simulink model "s32k344_mcb_sensorless_s32ct"  (R2024b)
settings: Solver=FixedStepAuto  StartTime=0.0  StopTime=20  RelTol=1e-3  EnableMultiTasking=on
PreLoadFcn:
  | % NXP_MBDT_S32K3 callback: DO NOT REMOVE
  | mbd_s32k3.common.nxp.model_callbacks.preLoadFcn();
  | 
  | s32k344Data;
  | mcbSensorlessData;
PostLoadFcn:
  | % NXP_MBDT_S32K3 callback: DO NOT REMOVE
  | mbd_s32k3.common.nxp.model_callbacks.postLoadFcn();
InitFcn:
  | % NXP_MBDT_S32K3 callback: DO NOT REMOVE
  | mbd_s32k3.common.nxp.model_callbacks.initFcn();
values from neighbouring files (symbols this model uses):
  PWM_DutyScale = 32768    [s32k344Data.m]
  PWM_Period = 8000    [s32k344Data.m]
  Ts_motor = T_pwm    (= 5e-05)    [s32k344Data.m]
  Ts_SerialIn = 0.1    [s32k344Data.m]
  Ts_SerialOut = 0.01    [s32k344Data.m]
  Ts_SysControl = 0.1    [mcbSensorlessData.m]
undefined symbols (not defined in the file or in its folder): inverter, LogicOutputId, pmsm, Value
libraries: mbd_s32k3_io_library x14, mbd_s32k3_cdd_library x4, simulink x4, mbd_s32k3_isr_library x1, mbd_s32k3_utility_library x1
(part 2 of 3)

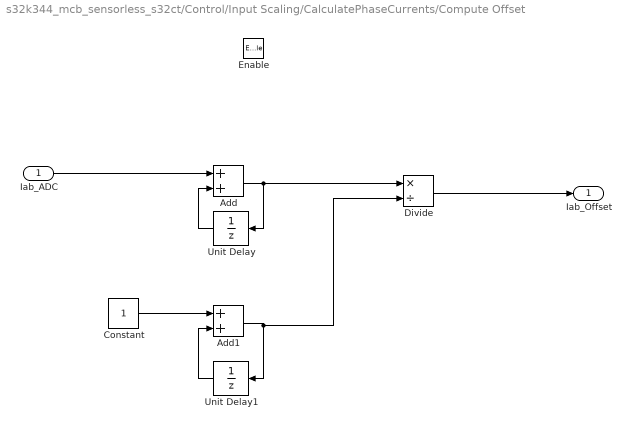
== system s32k344_mcb_sensorless_s32ct/Control/Input Scaling/CalculatePhaseCurrents/Compute Offset ==
  Iab_ADC : Inport
  Enable : EnablePort
  Add : Sum  RndMeth=Simplest  OutDataTypeStr=Inherit: Same as first input
  Add1 : Sum  RndMeth=Simplest  OutDataTypeStr=Inherit: Same as first input
  Constant : Constant  OutDataTypeStr=uint32  SampleTime=-1
  Divide : Product  Inputs=*/  RndMeth=Simplest  OutDataTypeStr=Inherit: Same as first input
  Unit Delay : UnitDelay  SampleTime=-1  HasFrameUpgradeWarning=on
  Unit Delay1 : UnitDelay  SampleTime=-1  HasFrameUpgradeWarning=on
  Iab_Offset : Outport
  wires:
  Iab_ADC/1 -> Add/1
  Unit Delay/1 -> Add/2
  Add/1 -> Divide/1, Unit Delay/1
  Constant/1 -> Add1/1
  Unit Delay1/1 -> Add1/2
  Add1/1 -> Divide/2, Unit Delay1/1
  Divide/1 -> Iab_Offset/1

== system s32k344_mcb_sensorless_s32ct/Control/SerialReceive/Variant Subsystem/CodeGeneration ==
  Constant : Constant  Value=8  OutDataTypeStr=Inherit: Inherit via back propagation
  Terminator : Terminator
  Uart : mbd_s32k3_cdd_library/Uart  api_func=Uart_AsyncReceive  channel=UartChannel_6  baudrate=UART_BAUDRATE_1200  transfer_type=UART_SEND  timeout=1  text=<binary blob, 3405 chars, not shown>
      settings: SourceProductName=CDD Blocks
  Data : Outport
  wires:
  Constant/1 -> Uart/1
  Uart/1 -> Data/1
  Uart/2 -> Terminator/1

== system s32k344_mcb_sensorless_s32ct/Control/SerialReceive/Variant Subsystem/Simulation ==
  Ground : Ground
  Data : Outport
  wires:
  Ground/1 -> Data/1

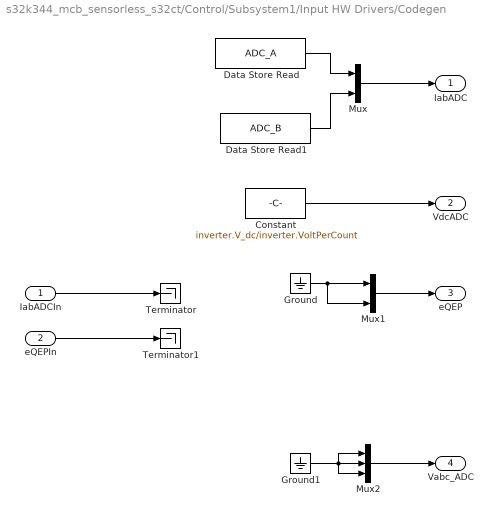
== system s32k344_mcb_sensorless_s32ct/Control/Subsystem1/Input HW Drivers/Codegen ==
  IabADCIn : Inport
  eQEPIn : Inport  Port=2
  Constant : Constant  Value=inverter.V_dc/inverter.VoltPerCount  OutDataTypeStr=uint16  SampleTime=-1
  Data Store Read : DataStoreRead  DataStoreName=ADC_A  IndexOptions=Index vector (dialog)  Indices=1  OutputSizes=1
  Data Store Read1 : DataStoreRead  DataStoreName=ADC_B  IndexOptions=Index vector (dialog)  Indices=1  OutputSizes=1
  Ground : Ground
  Ground1 : Ground
  Mux : Mux  Inputs=2
  Mux1 : Mux  Inputs=2
  Mux2 : Mux  Inputs=3
  Terminator : Terminator
  Terminator1 : Terminator
  IabADC : Outport
  VdcADC : Outport  Port=2
  eQEP : Outport  Port=3
  Vabc_ADC : Outport  Port=4
  wires:
  Ground/1 -> Mux1/2, Mux1/1
  Mux/1 -> IabADC/1
  Data Store Read1/1 -> Mux/2
  Constant/1 -> VdcADC/1
  Data Store Read/1 -> Mux/1
  Mux1/1 -> eQEP/1
  IabADCIn/1 -> Terminator/1
  eQEPIn/1 -> Terminator1/1
  Mux2/1 -> Vabc_ADC/1
  Ground1/1 -> Mux2/1, Mux2/3, Mux2/2

== system s32k344_mcb_sensorless_s32ct/Control/Subsystem1/Input HW Drivers/Sim ==
  IabADCIn : Inport
  eQEPIn : Inport  Port=2
  Constant : Constant  Value=inverter.V_dc/inverter.VoltPerCount  OutDataTypeStr=uint16  SampleTime=-1
  Ground : Ground
  IabADC : Outport
  VdcADC : Outport  Port=2
  Vabc_ADC : Outport  Port=3
  eQEP : Outport  Port=4
  wires:
  Constant/1 -> VdcADC/1
  Ground/1 -> Vabc_ADC/1
  IabADCIn/1 -> IabADC/1
  eQEPIn/1 -> eQEP/1

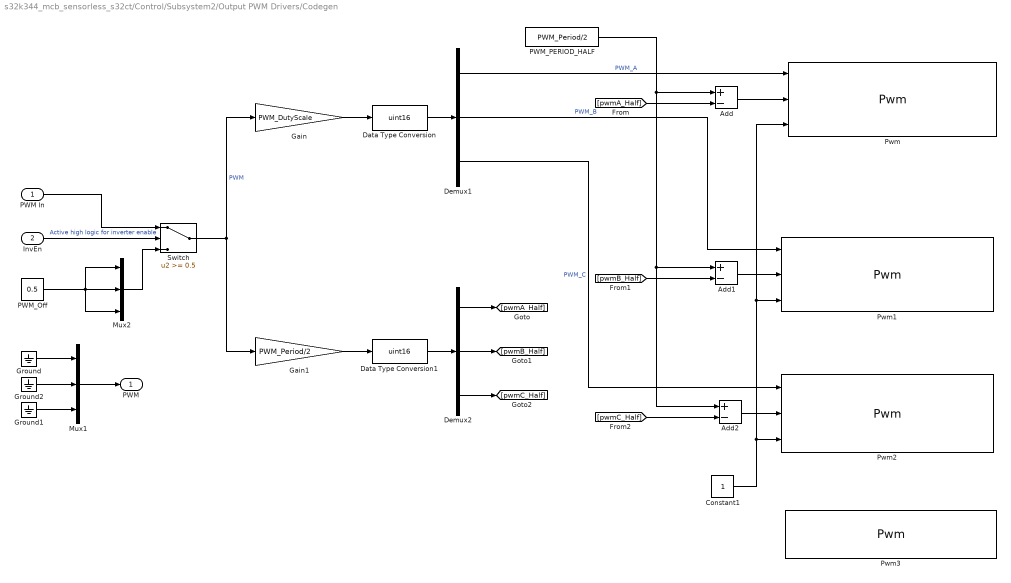
== system s32k344_mcb_sensorless_s32ct/Control/Subsystem2/Output PWM Drivers/Codegen ==
  PWM In : Inport
  InvEn : Inport  Port=2
  Add : Sum  Inputs=+-  OutDataTypeStr=uint16
  Add1 : Sum  Inputs=+-  OutDataTypeStr=uint16
  Add2 : Sum  Inputs=+-  OutDataTypeStr=uint16
  Constant1 : Constant  OutDataTypeStr=boolean  SampleTime=-1
  Data Type Conversion : DataTypeConversion  OutDataTypeStr=uint16  SaturateOnIntegerOverflow=off  RndMeth=Floor
  Data Type Conversion1 : DataTypeConversion  OutDataTypeStr=uint16  SaturateOnIntegerOverflow=off  RndMeth=Floor
  Demux1 : Demux  Outputs=3
  Demux2 : Demux  Outputs=3
  Gain : Gain  Gain=PWM_DutyScale  OutDataTypeStr=single
  Gain1 : Gain  Gain=PWM_Period/2  OutDataTypeStr=single
  Ground : Ground
  Ground1 : Ground
  Ground2 : Ground
  Mux1 : Mux  Inputs=3
  Mux2 : Mux  Inputs=3
  PWM_Off : Constant  Value=0.5  OutDataTypeStr=single
  PWM_PERIOD_HALF : Constant  Value=PWM_Period/2  OutDataTypeStr=uint16
  Pwm : mbd_s32k3_io_library/Pwm  api_func=Pwm_SetDutyPhaseShift  channel=PwmChannel_0  notification=PWM_RISING_EDGE  moduleId=PWM_EMIOS_INSTANCE_0  prescalerType=PWM_PRIMARY_PRESCALER  fault=PWM_FLEXPWM_0_FAULT_INPUT_0  text=|
      | CommonPublishedInformation - CommonPublishedInformation Pwm 
      | CommonPublishedInformation/ArReleaseMajorVersion - 4 
      | CommonPublishedInformation/ArReleaseMinorVersion - 7 
      | CommonPublishedInformation/ArReleaseRevisionVersion - 0 
      | CommonPublishedInformation/ModuleId - 121 
      | CommonPublishedInformation/SwMajorVersion - 4 
      | CommonPublishedInformation/SwMinorVersion - 0 
      | CommonPublishedInformation/SwPatchVersion - 0 
      | CommonPublishedInformation/VendorId - 43 
      | IMPLEMENTATION-CONFIG-VARIANT - VARIANT-POST-BUILD 
      | POST_BUILD_VARIANT_USED - true 
      | PwmChannel - PwmChannel_0 PwmChannel_1 PwmChannel_2 PwmChannel_3 
      | PwmChannel_0/Index - 0 
      | PwmChannel_0/PwmChannelId - 0 
      | PwmChannel_0/PwmDutycycleDefault - 16384 
      | PwmChannel_0/PwmHwChannel - /Pwm/Pwm/PwmChannelConfigSet/PwmEmios_0/PwmEmiosChannels_0 
      | PwmChannel_0/PwmIdleState - PWM_LOW 
      | PwmChannel_0/PwmMcuClockReferencePoint - /Mcu/Mcu/McuModuleConfiguration/McuClockSettingConfig_0/CORE_CLK 
      | PwmChannel_0/PwmPeriodDefault - 8000.0 
      | PwmChannel_0/PwmPeriodInTicks - true 
      | PwmChannel_0/PwmPolarity - PWM_HIGH 
      | PwmChannel_1/Index - 1 
      | PwmChannel_1/PwmChannelId - 1 
      | PwmChannel_1/PwmDutycycleDefault - 16384 
      | PwmChannel_1/PwmHwChannel - /Pwm/Pwm/PwmChannelConfigSet/PwmEmios_0/PwmEmiosChannels_1 
      | PwmChannel_1/PwmIdleState - PWM_LOW 
      | PwmChannel_1/PwmMcuClockReferencePoint - /Mcu/Mcu/McuModuleConfiguration/McuClockSettingConfig_0/CORE_CLK 
      | PwmChannel_1/PwmPeriodDefault - 8000.0 
      | PwmChannel_1/PwmPeriodInTicks - true 
      | PwmChannel_1/PwmPolarity - PWM_HIGH 
      | PwmChannel_2/Index - 2 
      | PwmChannel_2/PwmChannelId - 2 
      | PwmChannel_2/PwmDutycycleDefault - 16384 
      | PwmChannel_2/PwmHwChannel - /Pwm/Pwm/PwmChannelConfigSet/PwmEmios_0/PwmEmiosChannels_2 
      | PwmChannel_2/PwmIdleState - PWM_LOW 
      | PwmChannel_2/PwmMcuClockReferencePoint - /Mcu/Mcu/McuModuleConfiguration/McuClockSettingConfig_0/CORE_CLK 
      | PwmChannel_2/PwmPeriodDefault - 8000.0 
      | PwmChannel_2/PwmPeriodInTicks - true 
      | PwmChannel_2/PwmPolarity - PWM_HIGH 
      | PwmChannel_3/Index - 3 
      | PwmChannel_3/PwmChannelId - 3 
      | PwmChannel_3/PwmDutycycleDefault - 5 
      | PwmChannel_3/PwmHwChannel - /Pwm/Pwm/PwmChannelConfigSet/PwmEmios_0/PwmEmiosChannels_3 
      | PwmChannel_3/PwmIdleState - PWM_LOW 
      | PwmChannel_3/PwmMcuClockReferencePoint - /Mcu/Mcu/McuModuleConfiguration/McuClockSettingConfig_0/CORE_CLK 
      | PwmChannel_3/PwmPeriodDefault - 16000 
      | PwmChannel_3/PwmPeriodInTicks - true 
      | PwmChannel_3/PwmPolarity - PWM_HIGH 
      | PwmConfigurationOfOptApiServices - PwmConfigurationOfOptApiServices 
      | PwmConfigurationOfOptApiServices/PwmDeInitApi - false 
      | PwmConfigurationOfOptApiServices/PwmEmiosFastUpdateApi - true 
      | PwmConfigurationOfOptApiServices/PwmEnableMaskOutputs - false 
      | PwmConfigurationOfOptApiServices/PwmGetChannelStateApi - false 
      | PwmConfigurationOfOptApiServices/PwmGetOutputState - false 
      | PwmConfigurationOfOptApiServices/PwmSetChannelDeadTime - false 
      | PwmConfigurationOfOptApiServices/PwmSetChannelOutputApi - false 
      | PwmConfigurationOfOptApiServices/PwmSetCounterBusApi - false 
      | PwmConfigurationOfOptApiServices/PwmSetDutyCycle - true 
      | PwmConfigurationOfOptApiServices/PwmSetDutyCycle_NoUpdate - true 
      | PwmConfigurationOfOptApiServices/PwmSetDutyPhaseShift - true 
      | PwmConfigurationOfOptApiServices/PwmSetOutputToIdle - false 
      | PwmConfigurationOfOptApiServices/PwmSetPeriodAndDuty - false 
      | PwmConfigurationOfOptApiServices/PwmSetPeriodAndDuty_NoUpdate - false 
      | PwmConfigurationOfOptApiServices/PwmSetTriggerDelayApi - false 
      | PwmConfigurationOfOptApiServices/PwmVersionInfoApi - false 
      | PwmEmios - PwmEmios_0 
      | PwmEmios_0/Index - 0 
      | PwmEmios_0/PwmEmiosChannels - PwmEmiosChannels_0 PwmEmiosChannels_1 PwmEmiosChannels_2 PwmEmiosChannels_3 
      | PwmEmios_0/PwmEmiosChannels_0/EmiosChCounterBus - EMIOS_PWM_IP_BUS_BCD 
      | PwmEmios_0/PwmEmiosChannels_0/EmiosChDeadtime - 0 
      | PwmEmios_0/PwmEmiosChannels_0/EmiosChFlagGeneration - Trailing_Edge 
      | PwmEmios_0/PwmEmiosChannels_0/EmiosChFreeze - false 
      | PwmEmios_0/PwmEmiosChannels_0/EmiosChId - CH_1 
      | PwmEmios_0/PwmEmiosChannels_0/EmiosChInterrupt - EMIOS_PWM_IP_NOTIFICATION_DISABLED 
      | PwmEmios_0/PwmEmiosChannels_0/EmiosChMode - EMIOS_PWM_IP_MODE_OPWMB 
      | PwmEmios_0/PwmEmiosChannels_0/EmiosChOutputDisable - EMIOS_PWM_IP_OUTPUT_DISABLE_NONE 
      | PwmEmios_0/PwmEmiosChannels_0/EmiosChPhaseShift - 0 
      | PwmEmios_0/PwmEmiosChannels_0/EmiosChPrescaler - EMIOS_PWM_IP_CLOCK_DIV_1 
      | PwmEmios_0/PwmEmiosChannels_0/EmiosChPrescalerAlternate - EMIOS_PWM_IP_CLOCK_DIV_1 
      | PwmEmios_0/PwmEmiosChannels_0/EmiosChPrescalerSource - EMIOS_PWM_IP_PS_SRC_MODULE_CLOCK 
      | PwmEmios_0/PwmEmiosChannels_0/EmiosChTrigger - 0 
      | PwmEmios_0/PwmEmiosChannels_0/Index - 0 
      | PwmEmios_0/PwmEmiosChannels_0/PwmEmiosBusRef - /Mcl/Mcl/MclConfig/EmiosCommon_0/EmiosMclMasterBus_0 
      | PwmEmios_0/PwmEmiosChannels_1/EmiosChCounterBus - EMIOS_PWM_IP_BUS_BCD 
      | PwmEmios_0/PwmEmiosChannels_1/EmiosChDeadtime - 0 
      | PwmEmios_0/PwmEmiosChannels_1/EmiosChFlagGeneration - Trailing_Edge 
      | PwmEmios_0/PwmEmiosChannels_1/EmiosChFreeze - false 
      | PwmEmios_0/PwmEmiosChannels_1/EmiosChId - CH_2 
      | PwmEmios_0/PwmEmiosChannels_1/EmiosChInterrupt - EMIOS_PWM_IP_NOTIFICATION_DISABLED 
      | PwmEmios_0/PwmEmiosChannels_1/EmiosChMode - EMIOS_PWM_IP_MODE_OPWMB 
      | PwmEmios_0/PwmEmiosChannels_1/EmiosChOutputDisable - EMIOS_PWM_IP_OUTPUT_DISABLE_NONE 
      | PwmEmios_0/PwmEmiosChannels_1/EmiosChPhaseShift - 0 
      | PwmEmios_0/PwmEmiosChannels_1/EmiosChPrescaler - EMIOS_PWM_IP_CLOCK_DIV_1 
      | PwmEmios_0/PwmEmiosChannels_1/EmiosChPrescalerAlternate - EMIOS_PWM_IP_CLOCK_DIV_1 
      | PwmEmios_0/PwmEmiosChannels_1/EmiosChPrescalerSource - EMIOS_PWM_IP_PS_SRC_MODULE_CLOCK 
      | PwmEmios_0/PwmEmiosChannels_1/EmiosChTrigger - 0 
      | PwmEmios_0/PwmEmiosChannels_1/Index - 1 
      | PwmEmios_0/PwmEmiosChannels_1/PwmEmiosBusRef - /Mcl/Mcl/MclConfig/EmiosCommon_0/EmiosMclMasterBus_0 
      | PwmEmios_0/PwmEmiosChannels_2/EmiosChCounterBus - EMIOS_PWM_IP_BUS_BCD 
      | PwmEmios_0/PwmEmiosChannels_2/EmiosChDeadtime - 0 
      | PwmEmios_0/PwmEmiosChannels_2/EmiosChFlagGeneration - Trailing_Edge 
      | PwmEmios_0/PwmEmiosChannels_2/EmiosChFreeze - false 
      | PwmEmios_0/PwmEmiosChannels_2/EmiosChId - CH_3 
      | PwmEmios_0/PwmEmiosChannels_2/EmiosChInterrupt - EMIOS_PWM_IP_NOTIFICATION_DISABLED 
      | PwmEmios_0/PwmEmiosChannels_2/EmiosChMode - EMIOS_PWM_IP_MODE_OPWMB 
      | PwmEmios_0/PwmEmiosChannels_2/EmiosChOutputDisable - EMIOS_PWM_IP_OUTPUT_DISABLE_NONE 
      | PwmEmios_0/PwmEmiosChannels_2/EmiosChPhaseShift - 0 
      | PwmEmios_0/PwmEmiosChannels_2/EmiosChPrescaler - EMIOS_PWM_IP_CLOCK_DIV_1 
      | PwmEmios_0/PwmEmiosChannels_2/EmiosChPrescalerAlternate - EMIOS_PWM_IP_CLOCK_DIV_1 
      | PwmEmios_0/PwmEmiosChannels_2/EmiosChPrescalerSource - EMIOS_PWM_IP_PS_SRC_MODULE_CLOCK 
      | PwmEmios_0/PwmEmiosChannels_2/EmiosChTrigger - 0 
      | PwmEmios_0/PwmEmiosChannels_2/Index - 2 
      | PwmEmios_0/PwmEmiosChannels_2/PwmEmiosBusRef - /Mcl/Mcl/MclConfig/EmiosCommon_0/EmiosMclMasterBus_0 
      | PwmEmios_0/PwmEmiosChannels_3/EmiosChCounterBus - EMIOS_PWM_IP_BUS_A 
      | PwmEmios_0/PwmEmiosChannels_3/EmiosChDeadtime - 0 
      | PwmEmios_0/PwmEmiosChannels_3/EmiosChFlagGeneration - Trailing_Edge 
      | PwmEmios_0/PwmEmiosChannels_3/EmiosChFreeze - false 
      | PwmEmios_0/PwmEmiosChannels_3/EmiosChId - CH_4 
      | PwmEmios_0/PwmEmiosChannels_3/EmiosChInterrupt - EMIOS_PWM_IP_NOTIFICATION_DISABLED 
      | PwmEmios_0/PwmEmiosChannels_3/EmiosChMode - EMIOS_PWM_IP_MODE_OPWMB 
      | PwmEmios_0/PwmEmiosChannels_3/EmiosChOutputDisable - EMIOS_PWM_IP_OUTPUT_DISABLE_NONE 
      | PwmEmios_0/PwmEmiosChannels_3/EmiosChPhaseShift - 0 
      | PwmEmios_0/PwmEmiosChannels_3/EmiosChPrescaler - EMIOS_PWM_IP_CLOCK_DIV_1 
      | PwmEmios_0/PwmEmiosChannels_3/EmiosChPrescalerAlternate - EMIOS_PWM_IP_CLOCK_DIV_1 
      | PwmEmios_0/PwmEmiosChannels_3/EmiosChPrescalerSource - EMIOS_PWM_IP_PS_SRC_MODULE_CLOCK 
      | PwmEmios_0/PwmEmiosChannels_3/EmiosChTrigger - 0 
      | PwmEmios_0/PwmEmiosChannels_3/Index - 3 
      | PwmEmios_0/PwmEmiosChannels_3/PwmEmiosBusRef - /Mcl/Mcl/MclConfig/EmiosCommon_0/EmiosMclMasterBus_2 
      | PwmEmios_0/PwmHwInstance - Emios_0 
      | PwmEtpu - PwmChannelConfigSet 
      | PwmGeneral - PwmGeneral 
      | PwmGeneral/PwmDevErrorDetect - false 
      | PwmGeneral/PwmDutycycleUpdatedEndperiod - false 
      | PwmGeneral/PwmEnableDualClockMode - false 
      | PwmGeneral/PwmEnableUserModeSupport - false 
      | PwmGeneral/PwmFaultNotificationSupported - false 
      | PwmGeneral/PwmIndex - 0 
      | PwmGeneral/PwmMultiChannelSync - true 
      | PwmGeneral/PwmMultipartitionEnabled - false 
      | PwmGeneral/PwmNotificationSupported - false 
      | PwmGeneral/PwmPeriodUpdatedEndperiod - true
      settings: SourceProductName=IO Blocks
  Pwm1 : mbd_s32k3_io_library/Pwm  api_func=Pwm_SetDutyPhaseShift  channel=PwmChannel_1  notification=PWM_RISING_EDGE  moduleId=PWM_EMIOS_INSTANCE_0  prescalerType=PWM_PRIMARY_PRESCALER  fault=PWM_FLEXPWM_0_FAULT_INPUT_0  text=|
      | CommonPublishedInformation - CommonPublishedInformation Pwm 
      | CommonPublishedInformation/ArReleaseMajorVersion - 4 
      | CommonPublishedInformation/ArReleaseMinorVersion - 7 
      | CommonPublishedInformation/ArReleaseRevisionVersion - 0 
      | CommonPublishedInformation/ModuleId - 121 
      | CommonPublishedInformation/SwMajorVersion - 4 
      | CommonPublishedInformation/SwMinorVersion - 0 
      | CommonPublishedInformation/SwPatchVersion - 0 
      | CommonPublishedInformation/VendorId - 43 
      | IMPLEMENTATION-CONFIG-VARIANT - VARIANT-POST-BUILD 
      | POST_BUILD_VARIANT_USED - true 
      | PwmChannel - PwmChannel_0 PwmChannel_1 PwmChannel_2 PwmChannel_3 
      | PwmChannel_0/Index - 0 
      | PwmChannel_0/PwmChannelId - 0 
      | PwmChannel_0/PwmDutycycleDefault - 16384 
      | PwmChannel_0/PwmHwChannel - /Pwm/Pwm/PwmChannelConfigSet/PwmEmios_0/PwmEmiosChannels_0 
      | PwmChannel_0/PwmIdleState - PWM_LOW 
      | PwmChannel_0/PwmMcuClockReferencePoint - /Mcu/Mcu/McuModuleConfiguration/McuClockSettingConfig_0/CORE_CLK 
      | PwmChannel_0/PwmPeriodDefault - 8000.0 
      | PwmChannel_0/PwmPeriodInTicks - true 
      | PwmChannel_0/PwmPolarity - PWM_HIGH 
      | PwmChannel_1/Index - 1 
      | PwmChannel_1/PwmChannelId - 1 
      | PwmChannel_1/PwmDutycycleDefault - 16384 
      | PwmChannel_1/PwmHwChannel - /Pwm/Pwm/PwmChannelConfigSet/PwmEmios_0/PwmEmiosChannels_1 
      | PwmChannel_1/PwmIdleState - PWM_LOW 
      | PwmChannel_1/PwmMcuClockReferencePoint - /Mcu/Mcu/McuModuleConfiguration/McuClockSettingConfig_0/CORE_CLK 
      | PwmChannel_1/PwmPeriodDefault - 8000.0 
      | PwmChannel_1/PwmPeriodInTicks - true 
      | PwmChannel_1/PwmPolarity - PWM_HIGH 
      | PwmChannel_2/Index - 2 
      | PwmChannel_2/PwmChannelId - 2 
      | PwmChannel_2/PwmDutycycleDefault - 16384 
      | PwmChannel_2/PwmHwChannel - /Pwm/Pwm/PwmChannelConfigSet/PwmEmios_0/PwmEmiosChannels_2 
      | PwmChannel_2/PwmIdleState - PWM_LOW 
      | PwmChannel_2/PwmMcuClockReferencePoint - /Mcu/Mcu/McuModuleConfiguration/McuClockSettingConfig_0/CORE_CLK 
      | PwmChannel_2/PwmPeriodDefault - 8000.0 
      | PwmChannel_2/PwmPeriodInTicks - true 
      | PwmChannel_2/PwmPolarity - PWM_HIGH 
      | PwmChannel_3/Index - 3 
      | PwmChannel_3/PwmChannelId - 3 
      | PwmChannel_3/PwmDutycycleDefault - 5 
      | PwmChannel_3/PwmHwChannel - /Pwm/Pwm/PwmChannelConfigSet/PwmEmios_0/PwmEmiosChannels_3 
      | PwmChannel_3/PwmIdleState - PWM_LOW 
      | PwmChannel_3/PwmMcuClockReferencePoint - /Mcu/Mcu/McuModuleConfiguration/McuClockSettingConfig_0/CORE_CLK 
      | PwmChannel_3/PwmPeriodDefault - 16000 
      | PwmChannel_3/PwmPeriodInTicks - true 
      | PwmChannel_3/PwmPolarity - PWM_HIGH 
      | PwmConfigurationOfOptApiServices - PwmConfigurationOfOptApiServices 
      | PwmConfigurationOfOptApiServices/PwmDeInitApi - false 
      | PwmConfigurationOfOptApiServices/PwmEmiosFastUpdateApi - true 
      | PwmConfigurationOfOptApiServices/PwmEnableMaskOutputs - false 
      | PwmConfigurationOfOptApiServices/PwmGetChannelStateApi - false 
      | PwmConfigurationOfOptApiServices/PwmGetOutputState - false 
      | PwmConfigurationOfOptApiServices/PwmSetChannelDeadTime - false 
      | PwmConfigurationOfOptApiServices/PwmSetChannelOutputApi - false 
      | PwmConfigurationOfOptApiServices/PwmSetCounterBusApi - false 
      | PwmConfigurationOfOptApiServices/PwmSetDutyCycle - true 
      | PwmConfigurationOfOptApiServices/PwmSetDutyCycle_NoUpdate - true 
      | PwmConfigurationOfOptApiServices/PwmSetDutyPhaseShift - true 
      | PwmConfigurationOfOptApiServices/PwmSetOutputToIdle - false 
      | PwmConfigurationOfOptApiServices/PwmSetPeriodAndDuty - false 
      | PwmConfigurationOfOptApiServices/PwmSetPeriodAndDuty_NoUpdate - false 
      | PwmConfigurationOfOptApiServices/PwmSetTriggerDelayApi - false 
      | PwmConfigurationOfOptApiServices/PwmVersionInfoApi - false 
      | PwmEmios - PwmEmios_0 
      | PwmEmios_0/Index - 0 
      | PwmEmios_0/PwmEmiosChannels - PwmEmiosChannels_0 PwmEmiosChannels_1 PwmEmiosChannels_2 PwmEmiosChannels_3 
      | PwmEmios_0/PwmEmiosChannels_0/EmiosChCounterBus - EMIOS_PWM_IP_BUS_BCD 
      | PwmEmios_0/PwmEmiosChannels_0/EmiosChDeadtime - 0 
      | PwmEmios_0/PwmEmiosChannels_0/EmiosChFlagGeneration - Trailing_Edge 
      | PwmEmios_0/PwmEmiosChannels_0/EmiosChFreeze - false 
      | PwmEmios_0/PwmEmiosChannels_0/EmiosChId - CH_1 
      | PwmEmios_0/PwmEmiosChannels_0/EmiosChInterrupt - EMIOS_PWM_IP_NOTIFICATION_DISABLED 
      | PwmEmios_0/PwmEmiosChannels_0/EmiosChMode - EMIOS_PWM_IP_MODE_OPWMB 
      | PwmEmios_0/PwmEmiosChannels_0/EmiosChOutputDisable - EMIOS_PWM_IP_OUTPUT_DISABLE_NONE 
      | PwmEmios_0/PwmEmiosChannels_0/EmiosChPhaseShift - 0 
      | PwmEmios_0/PwmEmiosChannels_0/EmiosChPrescaler - EMIOS_PWM_IP_CLOCK_DIV_1 
      | PwmEmios_0/PwmEmiosChannels_0/EmiosChPrescalerAlternate - EMIOS_PWM_IP_CLOCK_DIV_1 
      | PwmEmios_0/PwmEmiosChannels_0/EmiosChPrescalerSource - EMIOS_PWM_IP_PS_SRC_MODULE_CLOCK 
      | PwmEmios_0/PwmEmiosChannels_0/EmiosChTrigger - 0 
      | PwmEmios_0/PwmEmiosChannels_0/Index - 0 
      | PwmEmios_0/PwmEmiosChannels_0/PwmEmiosBusRef - /Mcl/Mcl/MclConfig/EmiosCommon_0/EmiosMclMasterBus_0 
      | PwmEmios_0/PwmEmiosChannels_1/EmiosChCounterBus - EMIOS_PWM_IP_BUS_BCD 
      | PwmEmios_0/PwmEmiosChannels_1/EmiosChDeadtime - 0 
      | PwmEmios_0/PwmEmiosChannels_1/EmiosChFlagGeneration - Trailing_Edge 
      | PwmEmios_0/PwmEmiosChannels_1/EmiosChFreeze - false 
      | PwmEmios_0/PwmEmiosChannels_1/EmiosChId - CH_2 
      | PwmEmios_0/PwmEmiosChannels_1/EmiosChInterrupt - EMIOS_PWM_IP_NOTIFICATION_DISABLED 
      | PwmEmios_0/PwmEmiosChannels_1/EmiosChMode - EMIOS_PWM_IP_MODE_OPWMB 
      | PwmEmios_0/PwmEmiosChannels_1/EmiosChOutputDisable - EMIOS_PWM_IP_OUTPUT_DISABLE_NONE 
      | PwmEmios_0/PwmEmiosChannels_1/EmiosChPhaseShift - 0 
      | PwmEmios_0/PwmEmiosChannels_1/EmiosChPrescaler - EMIOS_PWM_IP_CLOCK_DIV_1 
      | PwmEmios_0/PwmEmiosChannels_1/EmiosChPrescalerAlternate - EMIOS_PWM_IP_CLOCK_DIV_1 
      | PwmEmios_0/PwmEmiosChannels_1/EmiosChPrescalerSource - EMIOS_PWM_IP_PS_SRC_MODULE_CLOCK 
      | PwmEmios_0/PwmEmiosChannels_1/EmiosChTrigger - 0 
      | PwmEmios_0/PwmEmiosChannels_1/Index - 1 
      | PwmEmios_0/PwmEmiosChannels_1/PwmEmiosBusRef - /Mcl/Mcl/MclConfig/EmiosCommon_0/EmiosMclMasterBus_0 
      | PwmEmios_0/PwmEmiosChannels_2/EmiosChCounterBus - EMIOS_PWM_IP_BUS_BCD 
      | PwmEmios_0/PwmEmiosChannels_2/EmiosChDeadtime - 0 
      | PwmEmios_0/PwmEmiosChannels_2/EmiosChFlagGeneration - Trailing_Edge 
      | PwmEmios_0/PwmEmiosChannels_2/EmiosChFreeze - false 
      | PwmEmios_0/PwmEmiosChannels_2/EmiosChId - CH_3 
      | PwmEmios_0/PwmEmiosChannels_2/EmiosChInterrupt - EMIOS_PWM_IP_NOTIFICATION_DISABLED 
      | PwmEmios_0/PwmEmiosChannels_2/EmiosChMode - EMIOS_PWM_IP_MODE_OPWMB 
      | PwmEmios_0/PwmEmiosChannels_2/EmiosChOutputDisable - EMIOS_PWM_IP_OUTPUT_DISABLE_NONE 
      | PwmEmios_0/PwmEmiosChannels_2/EmiosChPhaseShift - 0 
      | PwmEmios_0/PwmEmiosChannels_2/EmiosChPrescaler - EMIOS_PWM_IP_CLOCK_DIV_1 
      | PwmEmios_0/PwmEmiosChannels_2/EmiosChPrescalerAlternate - EMIOS_PWM_IP_CLOCK_DIV_1 
      | PwmEmios_0/PwmEmiosChannels_2/EmiosChPrescalerSource - EMIOS_PWM_IP_PS_SRC_MODULE_CLOCK 
      | PwmEmios_0/PwmEmiosChannels_2/EmiosChTrigger - 0 
      | PwmEmios_0/PwmEmiosChannels_2/Index - 2 
      | PwmEmios_0/PwmEmiosChannels_2/PwmEmiosBusRef - /Mcl/Mcl/MclConfig/EmiosCommon_0/EmiosMclMasterBus_0 
      | PwmEmios_0/PwmEmiosChannels_3/EmiosChCounterBus - EMIOS_PWM_IP_BUS_A 
      | PwmEmios_0/PwmEmiosChannels_3/EmiosChDeadtime - 0 
      | PwmEmios_0/PwmEmiosChannels_3/EmiosChFlagGeneration - Trailing_Edge 
      | PwmEmios_0/PwmEmiosChannels_3/EmiosChFreeze - false 
      | PwmEmios_0/PwmEmiosChannels_3/EmiosChId - CH_4 
      | PwmEmios_0/PwmEmiosChannels_3/EmiosChInterrupt - EMIOS_PWM_IP_NOTIFICATION_DISABLED 
      | PwmEmios_0/PwmEmiosChannels_3/EmiosChMode - EMIOS_PWM_IP_MODE_OPWMB 
      | PwmEmios_0/PwmEmiosChannels_3/EmiosChOutputDisable - EMIOS_PWM_IP_OUTPUT_DISABLE_NONE 
      | PwmEmios_0/PwmEmiosChannels_3/EmiosChPhaseShift - 0 
      | PwmEmios_0/PwmEmiosChannels_3/EmiosChPrescaler - EMIOS_PWM_IP_CLOCK_DIV_1 
      | PwmEmios_0/PwmEmiosChannels_3/EmiosChPrescalerAlternate - EMIOS_PWM_IP_CLOCK_DIV_1 
      | PwmEmios_0/PwmEmiosChannels_3/EmiosChPrescalerSource - EMIOS_PWM_IP_PS_SRC_MODULE_CLOCK 
      | PwmEmios_0/PwmEmiosChannels_3/EmiosChTrigger - 0 
      | PwmEmios_0/PwmEmiosChannels_3/Index - 3 
      | PwmEmios_0/PwmEmiosChannels_3/PwmEmiosBusRef - /Mcl/Mcl/MclConfig/EmiosCommon_0/EmiosMclMasterBus_2 
      | PwmEmios_0/PwmHwInstance - Emios_0 
      | PwmEtpu - PwmChannelConfigSet 
      | PwmGeneral - PwmGeneral 
      | PwmGeneral/PwmDevErrorDetect - false 
      | PwmGeneral/PwmDutycycleUpdatedEndperiod - false 
      | PwmGeneral/PwmEnableDualClockMode - false 
      | PwmGeneral/PwmEnableUserModeSupport - false 
      | PwmGeneral/PwmFaultNotificationSupported - false 
      | PwmGeneral/PwmIndex - 0 
      | PwmGeneral/PwmMultiChannelSync - true 
      | PwmGeneral/PwmMultipartitionEnabled - false 
      | PwmGeneral/PwmNotificationSupported - false 
      | PwmGeneral/PwmPeriodUpdatedEndperiod - true
      settings: SourceProductName=IO Blocks
  Pwm2 : mbd_s32k3_io_library/Pwm  api_func=Pwm_SetDutyPhaseShift  channel=PwmChannel_2  notification=PWM_RISING_EDGE  moduleId=PWM_EMIOS_INSTANCE_0  prescalerType=PWM_PRIMARY_PRESCALER  fault=PWM_FLEXPWM_0_FAULT_INPUT_0  text=|
      | CommonPublishedInformation - CommonPublishedInformation Pwm 
      | CommonPublishedInformation/ArReleaseMajorVersion - 4 
      | CommonPublishedInformation/ArReleaseMinorVersion - 7 
      | CommonPublishedInformation/ArReleaseRevisionVersion - 0 
      | CommonPublishedInformation/ModuleId - 121 
      | CommonPublishedInformation/SwMajorVersion - 4 
      | CommonPublishedInformation/SwMinorVersion - 0 
      | CommonPublishedInformation/SwPatchVersion - 0 
      | CommonPublishedInformation/VendorId - 43 
      | IMPLEMENTATION-CONFIG-VARIANT - VARIANT-POST-BUILD 
      | POST_BUILD_VARIANT_USED - true 
      | PwmChannel - PwmChannel_0 PwmChannel_1 PwmChannel_2 PwmChannel_3 
      | PwmChannel_0/Index - 0 
      | PwmChannel_0/PwmChannelId - 0 
      | PwmChannel_0/PwmDutycycleDefault - 16384 
      | PwmChannel_0/PwmHwChannel - /Pwm/Pwm/PwmChannelConfigSet/PwmEmios_0/PwmEmiosChannels_0 
      | PwmChannel_0/PwmIdleState - PWM_LOW 
      | PwmChannel_0/PwmMcuClockReferencePoint - /Mcu/Mcu/McuModuleConfiguration/McuClockSettingConfig_0/CORE_CLK 
      | PwmChannel_0/PwmPeriodDefault - 8000.0 
      | PwmChannel_0/PwmPeriodInTicks - true 
      | PwmChannel_0/PwmPolarity - PWM_HIGH 
      | PwmChannel_1/Index - 1 
      | PwmChannel_1/PwmChannelId - 1 
      | PwmChannel_1/PwmDutycycleDefault - 16384 
      | PwmChannel_1/PwmHwChannel - /Pwm/Pwm/PwmChannelConfigSet/PwmEmios_0/PwmEmiosChannels_1 
      | PwmChannel_1/PwmIdleState - PWM_LOW 
      | PwmChannel_1/PwmMcuClockReferencePoint - /Mcu/Mcu/McuModuleConfiguration/McuClockSettingConfig_0/CORE_CLK 
      | PwmChannel_1/PwmPeriodDefault - 8000.0 
      | PwmChannel_1/PwmPeriodInTicks - true 
      | PwmChannel_1/PwmPolarity - PWM_HIGH 
      | PwmChannel_2/Index - 2 
      | PwmChannel_2/PwmChannelId - 2 
      | PwmChannel_2/PwmDutycycleDefault - 16384 
      | PwmChannel_2/PwmHwChannel - /Pwm/Pwm/PwmChannelConfigSet/PwmEmios_0/PwmEmiosChannels_2 
      | PwmChannel_2/PwmIdleState - PWM_LOW 
      | PwmChannel_2/PwmMcuClockReferencePoint - /Mcu/Mcu/McuModuleConfiguration/McuClockSettingConfig_0/CORE_CLK 
      | PwmChannel_2/PwmPeriodDefault - 8000.0 
      | PwmChannel_2/PwmPeriodInTicks - true 
      | PwmChannel_2/PwmPolarity - PWM_HIGH 
      | PwmChannel_3/Index - 3 
      | PwmChannel_3/PwmChannelId - 3 
      | PwmChannel_3/PwmDutycycleDefault - 5 
      | PwmChannel_3/PwmHwChannel - /Pwm/Pwm/PwmChannelConfigSet/PwmEmios_0/PwmEmiosChannels_3 
      | PwmChannel_3/PwmIdleState - PWM_LOW 
      | PwmChannel_3/PwmMcuClockReferencePoint - /Mcu/Mcu/McuModuleConfiguration/McuClockSettingConfig_0/CORE_CLK 
      | PwmChannel_3/PwmPeriodDefault - 16000 
      | PwmChannel_3/PwmPeriodInTicks - true 
      | PwmChannel_3/PwmPolarity - PWM_HIGH 
      | PwmConfigurationOfOptApiServices - PwmConfigurationOfOptApiServices 
      | PwmConfigurationOfOptApiServices/PwmDeInitApi - false 
      | PwmConfigurationOfOptApiServices/PwmEmiosFastUpdateApi - true 
      | PwmConfigurationOfOptApiServices/PwmEnableMaskOutputs - false 
      | PwmConfigurationOfOptApiServices/PwmGetChannelStateApi - false 
      | PwmConfigurationOfOptApiServices/PwmGetOutputState - false 
      | PwmConfigurationOfOptApiServices/PwmSetChannelDeadTime - false 
      | PwmConfigurationOfOptApiServices/PwmSetChannelOutputApi - false 
      | PwmConfigurationOfOptApiServices/PwmSetCounterBusApi - false 
      | PwmConfigurationOfOptApiServices/PwmSetDutyCycle - true 
      | PwmConfigurationOfOptApiServices/PwmSetDutyCycle_NoUpdate - true 
      | PwmConfigurationOfOptApiServices/PwmSetDutyPhaseShift - true 
      | PwmConfigurationOfOptApiServices/PwmSetOutputToIdle - false 
      | PwmConfigurationOfOptApiServices/PwmSetPeriodAndDuty - false 
      | PwmConfigurationOfOptApiServices/PwmSetPeriodAndDuty_NoUpdate - false 
      | PwmConfigurationOfOptApiServices/PwmSetTriggerDelayApi - false 
      | PwmConfigurationOfOptApiServices/PwmVersionInfoApi - false 
      | PwmEmios - PwmEmios_0 
      | PwmEmios_0/Index - 0 
      | PwmEmios_0/PwmEmiosChannels - PwmEmiosChannels_0 PwmEmiosChannels_1 PwmEmiosChannels_2 PwmEmiosChannels_3 
      | PwmEmios_0/PwmEmiosChannels_0/EmiosChCounterBus - EMIOS_PWM_IP_BUS_BCD 
      | PwmEmios_0/PwmEmiosChannels_0/EmiosChDeadtime - 0 
      | PwmEmios_0/PwmEmiosChannels_0/EmiosChFlagGeneration - Trailing_Edge 
      | PwmEmios_0/PwmEmiosChannels_0/EmiosChFreeze - false 
      | PwmEmios_0/PwmEmiosChannels_0/EmiosChId - CH_1 
      | PwmEmios_0/PwmEmiosChannels_0/EmiosChInterrupt - EMIOS_PWM_IP_NOTIFICATION_DISABLED 
      | PwmEmios_0/PwmEmiosChannels_0/EmiosChMode - EMIOS_PWM_IP_MODE_OPWMB 
      | PwmEmios_0/PwmEmiosChannels_0/EmiosChOutputDisable - EMIOS_PWM_IP_OUTPUT_DISABLE_NONE 
      | PwmEmios_0/PwmEmiosChannels_0/EmiosChPhaseShift - 0 
      | PwmEmios_0/PwmEmiosChannels_0/EmiosChPrescaler - EMIOS_PWM_IP_CLOCK_DIV_1 
      | PwmEmios_0/PwmEmiosChannels_0/EmiosChPrescalerAlternate - EMIOS_PWM_IP_CLOCK_DIV_1 
      | PwmEmios_0/PwmEmiosChannels_0/EmiosChPrescalerSource - EMIOS_PWM_IP_PS_SRC_MODULE_CLOCK 
      | PwmEmios_0/PwmEmiosChannels_0/EmiosChTrigger - 0 
      | PwmEmios_0/PwmEmiosChannels_0/Index - 0 
      | PwmEmios_0/PwmEmiosChannels_0/PwmEmiosBusRef - /Mcl/Mcl/MclConfig/EmiosCommon_0/EmiosMclMasterBus_0 
      | PwmEmios_0/PwmEmiosChannels_1/EmiosChCounterBus - EMIOS_PWM_IP_BUS_BCD 
      | PwmEmios_0/PwmEmiosChannels_1/EmiosChDeadtime - 0 
      | PwmEmios_0/PwmEmiosChannels_1/EmiosChFlagGeneration - Trailing_Edge 
      | PwmEmios_0/PwmEmiosChannels_1/EmiosChFreeze - false 
      | PwmEmios_0/PwmEmiosChannels_1/EmiosChId - CH_2 
      | PwmEmios_0/PwmEmiosChannels_1/EmiosChInterrupt - EMIOS_PWM_IP_NOTIFICATION_DISABLED 
      | PwmEmios_0/PwmEmiosChannels_1/EmiosChMode - EMIOS_PWM_IP_MODE_OPWMB 
      | PwmEmios_0/PwmEmiosChannels_1/EmiosChOutputDisable - EMIOS_PWM_IP_OUTPUT_DISABLE_NONE 
      | PwmEmios_0/PwmEmiosChannels_1/EmiosChPhaseShift - 0 
      | PwmEmios_0/PwmEmiosChannels_1/EmiosChPrescaler - EMIOS_PWM_IP_CLOCK_DIV_1 
      | PwmEmios_0/PwmEmiosChannels_1/EmiosChPrescalerAlternate - EMIOS_PWM_IP_CLOCK_DIV_1 
      | PwmEmios_0/PwmEmiosChannels_1/EmiosChPrescalerSource - EMIOS_PWM_IP_PS_SRC_MODULE_CLOCK 
      | PwmEmios_0/PwmEmiosChannels_1/EmiosChTrigger - 0 
      | PwmEmios_0/PwmEmiosChannels_1/Index - 1 
      | PwmEmios_0/PwmEmiosChannels_1/PwmEmiosBusRef - /Mcl/Mcl/MclConfig/EmiosCommon_0/EmiosMclMasterBus_0 
      | PwmEmios_0/PwmEmiosChannels_2/EmiosChCounterBus - EMIOS_PWM_IP_BUS_BCD 
      | PwmEmios_0/PwmEmiosChannels_2/EmiosChDeadtime - 0 
      | PwmEmios_0/PwmEmiosChannels_2/EmiosChFlagGeneration - Trailing_Edge 
      | PwmEmios_0/PwmEmiosChannels_2/EmiosChFreeze - false 
      | PwmEmios_0/PwmEmiosChannels_2/EmiosChId - CH_3 
      | PwmEmios_0/PwmEmiosChannels_2/EmiosChInterrupt - EMIOS_PWM_IP_NOTIFICATION_DISABLED 
      | PwmEmios_0/PwmEmiosChannels_2/EmiosChMode - EMIOS_PWM_IP_MODE_OPWMB 
      | PwmEmios_0/PwmEmiosChannels_2/EmiosChOutputDisable - EMIOS_PWM_IP_OUTPUT_DISABLE_NONE 
      | PwmEmios_0/PwmEmiosChannels_2/EmiosChPhaseShift - 0 
      | PwmEmios_0/PwmEmiosChannels_2/EmiosChPrescaler - EMIOS_PWM_IP_CLOCK_DIV_1 
      | PwmEmios_0/PwmEmiosChannels_2/EmiosChPrescalerAlternate - EMIOS_PWM_IP_CLOCK_DIV_1 
      | PwmEmios_0/PwmEmiosChannels_2/EmiosChPrescalerSource - EMIOS_PWM_IP_PS_SRC_MODULE_CLOCK 
      | PwmEmios_0/PwmEmiosChannels_2/EmiosChTrigger - 0 
      | PwmEmios_0/PwmEmiosChannels_2/Index - 2 
      | PwmEmios_0/PwmEmiosChannels_2/PwmEmiosBusRef - /Mcl/Mcl/MclConfig/EmiosCommon_0/EmiosMclMasterBus_0 
      | PwmEmios_0/PwmEmiosChannels_3/EmiosChCounterBus - EMIOS_PWM_IP_BUS_A 
      | PwmEmios_0/PwmEmiosChannels_3/EmiosChDeadtime - 0 
      | PwmEmios_0/PwmEmiosChannels_3/EmiosChFlagGeneration - Trailing_Edge 
      | PwmEmios_0/PwmEmiosChannels_3/EmiosChFreeze - false 
      | PwmEmios_0/PwmEmiosChannels_3/EmiosChId - CH_4 
      | PwmEmios_0/PwmEmiosChannels_3/EmiosChInterrupt - EMIOS_PWM_IP_NOTIFICATION_DISABLED 
      | PwmEmios_0/PwmEmiosChannels_3/EmiosChMode - EMIOS_PWM_IP_MODE_OPWMB 
      | PwmEmios_0/PwmEmiosChannels_3/EmiosChOutputDisable - EMIOS_PWM_IP_OUTPUT_DISABLE_NONE 
      | PwmEmios_0/PwmEmiosChannels_3/EmiosChPhaseShift - 0 
      | PwmEmios_0/PwmEmiosChannels_3/EmiosChPrescaler - EMIOS_PWM_IP_CLOCK_DIV_1 
      | PwmEmios_0/PwmEmiosChannels_3/EmiosChPrescalerAlternate - EMIOS_PWM_IP_CLOCK_DIV_1 
      | PwmEmios_0/PwmEmiosChannels_3/EmiosChPrescalerSource - EMIOS_PWM_IP_PS_SRC_MODULE_CLOCK 
      | PwmEmios_0/PwmEmiosChannels_3/EmiosChTrigger - 0 
      | PwmEmios_0/PwmEmiosChannels_3/Index - 3 
      | PwmEmios_0/PwmEmiosChannels_3/PwmEmiosBusRef - /Mcl/Mcl/MclConfig/EmiosCommon_0/EmiosMclMasterBus_2 
      | PwmEmios_0/PwmHwInstance - Emios_0 
      | PwmEtpu - PwmChannelConfigSet 
      | PwmGeneral - PwmGeneral 
      | PwmGeneral/PwmDevErrorDetect - false 
      | PwmGeneral/PwmDutycycleUpdatedEndperiod - false 
      | PwmGeneral/PwmEnableDualClockMode - false 
      | PwmGeneral/PwmEnableUserModeSupport - false 
      | PwmGeneral/PwmFaultNotificationSupported - false 
      | PwmGeneral/PwmIndex - 0 
      | PwmGeneral/PwmMultiChannelSync - true 
      | PwmGeneral/PwmMultipartitionEnabled - false 
      | PwmGeneral/PwmNotificationSupported - false 
      | PwmGeneral/PwmPeriodUpdatedEndperiod - true
      settings: SourceProductName=IO Blocks
  Pwm3 : mbd_s32k3_io_library/Pwm  api_func=Pwm_SyncUpdate  channel=PwmChannel_0  notification=PWM_RISING_EDGE  moduleId=PWM_EMIOS_INSTANCE_0  prescalerType=PWM_PRIMARY_PRESCALER  fault=PWM_FLEXPWM_0_FAULT_INPUT_0  text=|
      | CommonPublishedInformation - CommonPublishedInformation Pwm 
      | CommonPublishedInformation/ArReleaseMajorVersion - 4 
      | CommonPublishedInformation/ArReleaseMinorVersion - 7 
      | CommonPublishedInformation/ArReleaseRevisionVersion - 0 
      | CommonPublishedInformation/ModuleId - 121 
      | CommonPublishedInformation/SwMajorVersion - 4 
      | CommonPublishedInformation/SwMinorVersion - 0 
      | CommonPublishedInformation/SwPatchVersion - 0 
      | CommonPublishedInformation/VendorId - 43 
      | IMPLEMENTATION-CONFIG-VARIANT - VARIANT-POST-BUILD 
      | POST_BUILD_VARIANT_USED - true 
      | PwmChannel - PwmChannel_0 PwmChannel_1 PwmChannel_2 PwmChannel_3 
      | PwmChannel_0/Index - 0 
      | PwmChannel_0/PwmChannelId - 0 
      | PwmChannel_0/PwmDutycycleDefault - 16384 
      | PwmChannel_0/PwmHwChannel - /Pwm/Pwm/PwmChannelConfigSet/PwmEmios_0/PwmEmiosChannels_0 
      | PwmChannel_0/PwmIdleState - PWM_LOW 
      | PwmChannel_0/PwmMcuClockReferencePoint - /Mcu/Mcu/McuModuleConfiguration/McuClockSettingConfig_0/CORE_CLK 
      | PwmChannel_0/PwmPeriodDefault - 8000.0 
      | PwmChannel_0/PwmPeriodInTicks - true 
      | PwmChannel_0/PwmPolarity - PWM_HIGH 
      | PwmChannel_1/Index - 1 
      | PwmChannel_1/PwmChannelId - 1 
      | PwmChannel_1/PwmDutycycleDefault - 16384 
      | PwmChannel_1/PwmHwChannel - /Pwm/Pwm/PwmChannelConfigSet/PwmEmios_0/PwmEmiosChannels_1 
      | PwmChannel_1/PwmIdleState - PWM_LOW 
      | PwmChannel_1/PwmMcuClockReferencePoint - /Mcu/Mcu/McuModuleConfiguration/McuClockSettingConfig_0/CORE_CLK 
      | PwmChannel_1/PwmPeriodDefault - 8000.0 
      | PwmChannel_1/PwmPeriodInTicks - true 
      | PwmChannel_1/PwmPolarity - PWM_HIGH 
      | PwmChannel_2/Index - 2 
      | PwmChannel_2/PwmChannelId - 2 
      | PwmChannel_2/PwmDutycycleDefault - 16384 
      | PwmChannel_2/PwmHwChannel - /Pwm/Pwm/PwmChannelConfigSet/PwmEmios_0/PwmEmiosChannels_2 
      | PwmChannel_2/PwmIdleState - PWM_LOW 
      | PwmChannel_2/PwmMcuClockReferencePoint - /Mcu/Mcu/McuModuleConfiguration/McuClockSettingConfig_0/CORE_CLK 
      | PwmChannel_2/PwmPeriodDefault - 8000.0 
      | PwmChannel_2/PwmPeriodInTicks - true 
      | PwmChannel_2/PwmPolarity - PWM_HIGH 
      | PwmChannel_3/Index - 3 
      | PwmChannel_3/PwmChannelId - 3 
      | PwmChannel_3/PwmDutycycleDefault - 5 
      | PwmChannel_3/PwmHwChannel - /Pwm/Pwm/PwmChannelConfigSet/PwmEmios_0/PwmEmiosChannels_3 
      | PwmChannel_3/PwmIdleState - PWM_LOW 
      | PwmChannel_3/PwmMcuClockReferencePoint - /Mcu/Mcu/McuModuleConfiguration/McuClockSettingConfig_0/CORE_CLK 
      | PwmChannel_3/PwmPeriodDefault - 16000 
      | PwmChannel_3/PwmPeriodInTicks - true 
      | PwmChannel_3/PwmPolarity - PWM_HIGH 
      | PwmConfigurationOfOptApiServices - PwmConfigurationOfOptApiServices 
      | PwmConfigurationOfOptApiServices/PwmDeInitApi - false 
      | PwmConfigurationOfOptApiServices/PwmEmiosFastUpdateApi - true 
      | PwmConfigurationOfOptApiServices/PwmEnableMaskOutputs - false 
      | PwmConfigurationOfOptApiServices/PwmGetChannelStateApi - false 
      | PwmConfigurationOfOptApiServices/PwmGetOutputState - false 
      | PwmConfigurationOfOptApiServices/PwmSetChannelDeadTime - false 
      | PwmConfigurationOfOptApiServices/PwmSetChannelOutputApi - false 
      | PwmConfigurationOfOptApiServices/PwmSetCounterBusApi - false 
      | PwmConfigurationOfOptApiServices/PwmSetDutyCycle - true 
      | PwmConfigurationOfOptApiServices/PwmSetDutyCycle_NoUpdate - true 
      | PwmConfigurationOfOptApiServices/PwmSetDutyPhaseShift - true 
      | PwmConfigurationOfOptApiServices/PwmSetOutputToIdle - false 
      | PwmConfigurationOfOptApiServices/PwmSetPeriodAndDuty - false 
      | PwmConfigurationOfOptApiServices/PwmSetPeriodAndDuty_NoUpdate - false 
      | PwmConfigurationOfOptApiServices/PwmSetTriggerDelayApi - false 
      | PwmConfigurationOfOptApiServices/PwmVersionInfoApi - false 
      | PwmEmios - PwmEmios_0 
      | PwmEmios_0/Index - 0 
      | PwmEmios_0/PwmEmiosChannels - PwmEmiosChannels_0 PwmEmiosChannels_1 PwmEmiosChannels_2 PwmEmiosChannels_3 
      | PwmEmios_0/PwmEmiosChannels_0/EmiosChCounterBus - EMIOS_PWM_IP_BUS_BCD 
      | PwmEmios_0/PwmEmiosChannels_0/EmiosChDeadtime - 0 
      | PwmEmios_0/PwmEmiosChannels_0/EmiosChFlagGeneration - Trailing_Edge 
      | PwmEmios_0/PwmEmiosChannels_0/EmiosChFreeze - false 
      | PwmEmios_0/PwmEmiosChannels_0/EmiosChId - CH_1 
      | PwmEmios_0/PwmEmiosChannels_0/EmiosChInterrupt - EMIOS_PWM_IP_NOTIFICATION_DISABLED 
      | PwmEmios_0/PwmEmiosChannels_0/EmiosChMode - EMIOS_PWM_IP_MODE_OPWMB 
      | PwmEmios_0/PwmEmiosChannels_0/EmiosChOutputDisable - EMIOS_PWM_IP_OUTPUT_DISABLE_NONE 
      | PwmEmios_0/PwmEmiosChannels_0/EmiosChPhaseShift - 0 
      | PwmEmios_0/PwmEmiosChannels_0/EmiosChPrescaler - EMIOS_PWM_IP_CLOCK_DIV_1 
      | PwmEmios_0/PwmEmiosChannels_0/EmiosChPrescalerAlternate - EMIOS_PWM_IP_CLOCK_DIV_1 
      | PwmEmios_0/PwmEmiosChannels_0/EmiosChPrescalerSource - EMIOS_PWM_IP_PS_SRC_MODULE_CLOCK 
      | PwmEmios_0/PwmEmiosChannels_0/EmiosChTrigger - 0 
      | PwmEmios_0/PwmEmiosChannels_0/Index - 0 
      | PwmEmios_0/PwmEmiosChannels_0/PwmEmiosBusRef - /Mcl/Mcl/MclConfig/EmiosCommon_0/EmiosMclMasterBus_0 
      | PwmEmios_0/PwmEmiosChannels_1/EmiosChCounterBus - EMIOS_PWM_IP_BUS_BCD 
      | PwmEmios_0/PwmEmiosChannels_1/EmiosChDeadtime - 0 
      | PwmEmios_0/PwmEmiosChannels_1/EmiosChFlagGeneration - Trailing_Edge 
      | PwmEmios_0/PwmEmiosChannels_1/EmiosChFreeze - false 
      | PwmEmios_0/PwmEmiosChannels_1/EmiosChId - CH_2 
      | PwmEmios_0/PwmEmiosChannels_1/EmiosChInterrupt - EMIOS_PWM_IP_NOTIFICATION_DISABLED 
      | PwmEmios_0/PwmEmiosChannels_1/EmiosChMode - EMIOS_PWM_IP_MODE_OPWMB 
      | PwmEmios_0/PwmEmiosChannels_1/EmiosChOutputDisable - EMIOS_PWM_IP_OUTPUT_DISABLE_NONE 
      | PwmEmios_0/PwmEmiosChannels_1/EmiosChPhaseShift - 0 
      | PwmEmios_0/PwmEmiosChannels_1/EmiosChPrescaler - EMIOS_PWM_IP_CLOCK_DIV_1 
      | PwmEmios_0/PwmEmiosChannels_1/EmiosChPrescalerAlternate - EMIOS_PWM_IP_CLOCK_DIV_1 
      | PwmEmios_0/PwmEmiosChannels_1/EmiosChPrescalerSource - EMIOS_PWM_IP_PS_SRC_MODULE_CLOCK 
      | PwmEmios_0/PwmEmiosChannels_1/EmiosChTrigger - 0 
      | PwmEmios_0/PwmEmiosChannels_1/Index - 1 
      | PwmEmios_0/PwmEmiosChannels_1/PwmEmiosBusRef - /Mcl/Mcl/MclConfig/EmiosCommon_0/EmiosMclMasterBus_0 
      | PwmEmios_0/PwmEmiosChannels_2/EmiosChCounterBus - EMIOS_PWM_IP_BUS_BCD 
      | PwmEmios_0/PwmEmiosChannels_2/EmiosChDeadtime - 0 
      | PwmEmios_0/PwmEmiosChannels_2/EmiosChFlagGeneration - Trailing_Edge 
      | PwmEmios_0/PwmEmiosChannels_2/EmiosChFreeze - false 
      | PwmEmios_0/PwmEmiosChannels_2/EmiosChId - CH_3 
      | PwmEmios_0/PwmEmiosChannels_2/EmiosChInterrupt - EMIOS_PWM_IP_NOTIFICATION_DISABLED 
      | PwmEmios_0/PwmEmiosChannels_2/EmiosChMode - EMIOS_PWM_IP_MODE_OPWMB 
      | PwmEmios_0/PwmEmiosChannels_2/EmiosChOutputDisable - EMIOS_PWM_IP_OUTPUT_DISABLE_NONE 
      | PwmEmios_0/PwmEmiosChannels_2/EmiosChPhaseShift - 0 
      | PwmEmios_0/PwmEmiosChannels_2/EmiosChPrescaler - EMIOS_PWM_IP_CLOCK_DIV_1 
      | PwmEmios_0/PwmEmiosChannels_2/EmiosChPrescalerAlternate - EMIOS_PWM_IP_CLOCK_DIV_1 
      | PwmEmios_0/PwmEmiosChannels_2/EmiosChPrescalerSource - EMIOS_PWM_IP_PS_SRC_MODULE_CLOCK 
      | PwmEmios_0/PwmEmiosChannels_2/EmiosChTrigger - 0 
      | PwmEmios_0/PwmEmiosChannels_2/Index - 2 
      | PwmEmios_0/PwmEmiosChannels_2/PwmEmiosBusRef - /Mcl/Mcl/MclConfig/EmiosCommon_0/EmiosMclMasterBus_0 
      | PwmEmios_0/PwmEmiosChannels_3/EmiosChCounterBus - EMIOS_PWM_IP_BUS_A 
      | PwmEmios_0/PwmEmiosChannels_3/EmiosChDeadtime - 0 
      | PwmEmios_0/PwmEmiosChannels_3/EmiosChFlagGeneration - Trailing_Edge 
      | PwmEmios_0/PwmEmiosChannels_3/EmiosChFreeze - false 
      | PwmEmios_0/PwmEmiosChannels_3/EmiosChId - CH_4 
      | PwmEmios_0/PwmEmiosChannels_3/EmiosChInterrupt - EMIOS_PWM_IP_NOTIFICATION_DISABLED 
      | PwmEmios_0/PwmEmiosChannels_3/EmiosChMode - EMIOS_PWM_IP_MODE_OPWMB 
      | PwmEmios_0/PwmEmiosChannels_3/EmiosChOutputDisable - EMIOS_PWM_IP_OUTPUT_DISABLE_NONE 
      | PwmEmios_0/PwmEmiosChannels_3/EmiosChPhaseShift - 0 
      | PwmEmios_0/PwmEmiosChannels_3/EmiosChPrescaler - EMIOS_PWM_IP_CLOCK_DIV_1 
      | PwmEmios_0/PwmEmiosChannels_3/EmiosChPrescalerAlternate - EMIOS_PWM_IP_CLOCK_DIV_1 
      | PwmEmios_0/PwmEmiosChannels_3/EmiosChPrescalerSource - EMIOS_PWM_IP_PS_SRC_MODULE_CLOCK 
      | PwmEmios_0/PwmEmiosChannels_3/EmiosChTrigger - 0 
      | PwmEmios_0/PwmEmiosChannels_3/Index - 3 
      | PwmEmios_0/PwmEmiosChannels_3/PwmEmiosBusRef - /Mcl/Mcl/MclConfig/EmiosCommon_0/EmiosMclMasterBus_2 
      | PwmEmios_0/PwmHwInstance - Emios_0 
      | PwmEtpu - PwmChannelConfigSet 
      | PwmGeneral - PwmGeneral 
      | PwmGeneral/PwmDevErrorDetect - false 
      | PwmGeneral/PwmDutycycleUpdatedEndperiod - false 
      | PwmGeneral/PwmEnableDualClockMode - false 
      | PwmGeneral/PwmEnableUserModeSupport - false 
      | PwmGeneral/PwmFaultNotificationSupported - false 
      | PwmGeneral/PwmIndex - 0 
      | PwmGeneral/PwmMultiChannelSync - true 
      | PwmGeneral/PwmMultipartitionEnabled - false 
      | PwmGeneral/PwmNotificationSupported - false 
      | PwmGeneral/PwmPeriodUpdatedEndperiod - true
      settings: SourceProductName=IO Blocks
  Switch : Switch  Threshold=0.5  OutDataTypeStr=single  SaturateOnIntegerOverflow=off  InputSameDT=off
  PWM : Outport
  wires:
  Mux1/1 -> PWM/1
  Ground2/1 -> Mux1/2
  Ground1/1 -> Mux1/3
  Ground/1 -> Mux1/1
  Mux2/1 -> Switch/3
  PWM_Off/1 -> Mux2/3, Mux2/1, Mux2/2
  InvEn/1 -> Switch/2  "Active high logic for inverter enable"
  PWM In/1 -> Switch/1
  Add/1 -> Pwm/2
  [pwmA_Half] -> Add/2
  Data Type Conversion1/1 -> Demux2/1
  Demux1/2 -> Pwm1/1  "PWM_B"
  [pwmB_Half] -> Add1/2
  Gain/1 -> Data Type Conversion/1
  Add2/1 -> Pwm2/2
  Demux2/2 -> [pwmB_Half]
  Constant1/1 -> Pwm2/3, Pwm1/3, Pwm/3
  PWM_PERIOD_HALF/1 -> Add/1, Add1/1, Add2/1
  Demux1/1 -> Pwm/1  "PWM_A"
  Demux2/1 -> [pwmA_Half]
  Data Type Conversion/1 -> Demux1/1
  [pwmC_Half] -> Add2/2
  Add1/1 -> Pwm1/2
  Gain1/1 -> Data Type Conversion1/1
  Demux2/3 -> [pwmC_Half]
  Demux1/3 -> Pwm2/1  "PWM_C"
  Switch/1 -> Gain1/1, Gain/1  "PWM"

== system s32k344_mcb_sensorless_s32ct/Control/Subsystem2/Output PWM Drivers/Sim ==
  PWM In : Inport
  InvEn : Inport  Port=2
  Data Type Duplicate : DataTypeDuplicate
  Mux2 : Mux  Inputs=3
  Switch : Switch  Threshold=0.5  RndMeth=Simplest  SaturateOnIntegerOverflow=off  InputSameDT=off
  stop : Constant  Value=0  OutDataTypeStr=Inherit: Inherit via back propagation
  PWM : Outport
  wires:
  PWM In/1 -> Data Type Duplicate/1, Switch/1  "PWM Duty Cycles"
  Mux2/1 -> Switch/3
  Switch/1 -> PWM/1
  stop/1 -> Data Type Duplicate/2, Mux2/1, Mux2/3, Mux2/2
  InvEn/1 -> Switch/2

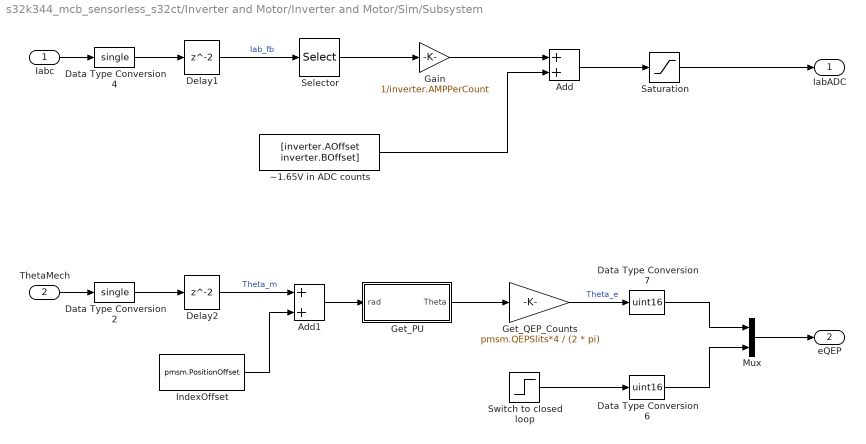
== system s32k344_mcb_sensorless_s32ct/Inverter and Motor/Inverter and Motor/Sim/Subsystem ==
  Iabc : Inport
  ThetaMech : Inport  Port=2
  Add : Sum  RndMeth=Simplest  OutDataTypeStr=Inherit: Same as first input
  Add1 : Sum  RndMeth=Simplest
  Data Type Conversion2 : DataTypeConversion  OutDataTypeStr=single  RndMeth=Simplest  SaturateOnIntegerOverflow=off
  Data Type Conversion4 : DataTypeConversion  OutDataTypeStr=single  RndMeth=Simplest  SaturateOnIntegerOverflow=off
  Data Type Conversion6 : DataTypeConversion  OutDataTypeStr=uint16  RndMeth=Simplest  SaturateOnIntegerOverflow=off
  Data Type Conversion7 : DataTypeConversion  OutDataTypeStr=uint16  RndMeth=Simplest  SaturateOnIntegerOverflow=off
  Delay1 : Delay
  Delay2 : Delay
  Gain : Gain  Gain=1/inverter.AMPPerCount  OutDataTypeStr=int16
  "Get_PU " : Subsystem
  Get_QEP_Counts : Gain  Gain=pmsm.QEPSlits*4 / (2 * pi)  OutDataTypeStr=uint16  RndMeth=Simplest
  IndexOffset : Constant  Value=pmsm.PositionOffset  OutDataTypeStr=single  SampleTime=-1
  Mux : Mux  Inputs=2
  Saturation : Saturate  UpperLimit=inverter.MaxADCCnt  LowerLimit=0  OutDataTypeStr=uint16  RndMeth=Simplest
  Selector : Selector  InputPortWidth=3  IndexOptions=Index vector (dialog)  Indices=[1 2]  OutputSizes=1
  "Switch to closed loop " : Step  Time=0.1  SampleTime=Ts_motor
  ~1.65V in ADC counts : Constant  Value=[inverter.AOffset inverter.BOffset]  OutDataTypeStr=uint16  SampleTime=-1
  IabADC : Outport
  eQEP : Outport  Port=2
  wires:
  "Switch to closed loop "/1 -> Data Type Conversion6/1
  Iabc/1 -> Data Type Conversion4/1
  Get_QEP_Counts/1 -> Data Type Conversion7/1  "Theta_e"
  Mux/1 -> eQEP/1
  Data Type Conversion6/1 -> Mux/2
  Delay1/1 -> Selector/1  "Iab_fb"
  "Get_PU "/1(Theta) -> Get_QEP_Counts/1
  IndexOffset/1 -> Add1/2
  Data Type Conversion7/1 -> Mux/1
  Data Type Conversion2/1 -> Delay2/1
  Data Type Conversion4/1 -> Delay1/1
  ThetaMech/1 -> Data Type Conversion2/1
  Saturation/1 -> IabADC/1
  Selector/1 -> Gain/1
  Gain/1 -> Add/1
  ~1.65V in ADC counts/1 -> Add/2
  Add/1 -> Saturation/1
  Delay2/1 -> Add1/1  "Theta_m"
  Add1/1 -> "Get_PU "/1(rad)

== system s32k344_mcb_sensorless_s32ct/Control/HW INT/CodeGeneration/ADC_INT/ADC_IRQHandler ==
  function : TriggerPort  TriggerType=function-call  VariantControl=(inherit)
  Adc : mbd_s32k3_io_library/Adc  Priority=0  api_func=Adc_CtuReadFifoData  hw_unit=AdcHwUnit_0  group=Adc0Group_0  channel=PHB_I  threshold_control=No ADC threshold control configured  power_state=ADC_FULL_POWER  ctu_unit=BctuHwUnit_0  ctu_trigger=AdcHwTrigger_0  ctu_fifo_idx=BctuResultFifos_0  text=<binary blob, 26323 chars, not shown>
      settings: SourceProductName=IO Blocks
  Demux : Demux
  Fault Detection : Subsystem  TreatAsAtomicUnit=on
      settings: RTWSystemCode=Nonreusable function
  Function-Call Generator : simulink/Ports & Subsystems/Function-Call Generator  Priority=1  sample_time=-1  numberOfIterations=1  DisallowWideOutput=off
  Mux : Mux  Inputs=2
  Terminator : Terminator
  ADC_Event : Outport
  ADC_Res : Outport  Port=2
  wires:
  Function-Call Generator/1 -> ADC_Event/1
  Mux/1 -> ADC_Res/1
  Demux/2 -> Mux/2  "ADC_IA"
  Demux/1 -> Mux/1  "ADC_IB"
  Demux/4 -> Terminator/1
  Demux/3 -> Fault Detection/1(VDC)  "ADC_VDC"
  Adc/1 -> Demux/1

== system s32k344_mcb_sensorless_s32ct/Control/Input Scaling/Calculate Phase Currents/Automatic offset calibration/Compute Offset ==
  Iab_ADC : Inport
  Enable : EnablePort
  Add : Sum  RndMeth=Simplest  OutDataTypeStr=Inherit: Same as first input
  Add1 : Sum  RndMeth=Simplest  OutDataTypeStr=Inherit: Same as first input
  Constant : Constant  OutDataTypeStr=uint32  SampleTime=50e-6
  Divide : Product  Inputs=*/  RndMeth=Simplest  OutDataTypeStr=Inherit: Same as first input
  Unit Delay : UnitDelay  SampleTime=-1  HasFrameUpgradeWarning=on
  Unit Delay1 : UnitDelay  SampleTime=-1  HasFrameUpgradeWarning=on
  Iab_Offset : Outport
  wires:
  Iab_ADC/1 -> Add/1
  Unit Delay/1 -> Add/2
  Add/1 -> Divide/1, Unit Delay/1
  Constant/1 -> Add1/1
  Unit Delay1/1 -> Add1/2
  Add1/1 -> Divide/2, Unit Delay1/1
  Divide/1 -> Iab_Offset/1

== system s32k344_mcb_sensorless_s32ct/Inverter and Motor/Inverter and Motor/Sim/Subsystem/Get_PU  ==
  rad : Inport
  Constant2 : Constant  Value=2*pi  OutDataTypeStr=single  SampleTime=-1
  Mod : Math  Operator=mod
  Theta : Outport  VectorParamsAs1DForOutWhenUnconnected=off
  wires:
  Constant2/1 -> Mod/2
  rad/1 -> Mod/1
  Mod/1 -> Theta/1
